simulink subsystem "out_of_wave"  (R2025b)
settings: Solver=VariableStepAuto  StartTime=0.0  StopTime=10.0  RelTol=1e-3
settings Model: Creator=sanborkl  LastModifiedBy=jdcjdb

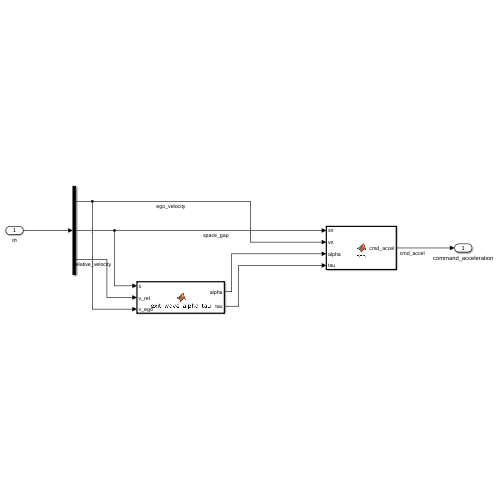
[thumbnail: Simulink's stored preview of the top-level diagram]
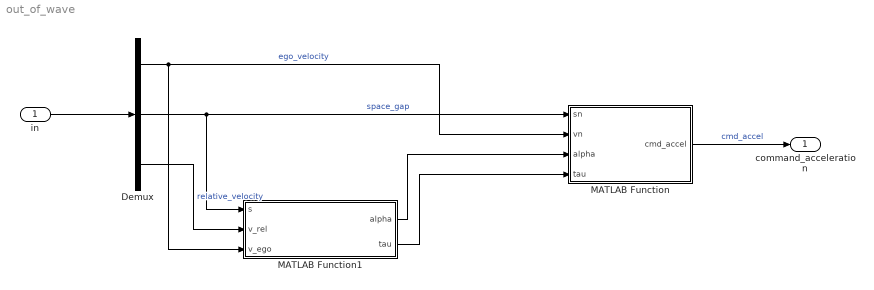
== system out_of_wave ==
  in : Inport
  Demux : Demux  Outputs=3
  MATLAB Function : MATLAB Function  TreatAsAtomicUnit=on
  MATLAB Function1 : MATLAB Function  TreatAsAtomicUnit=on
  command_acceleration : Outport
  wires:
  MATLAB Function1/1(alpha) -> MATLAB Function/3(alpha)
  MATLAB Function1/2(tau) -> MATLAB Function/4(tau)
  in/1 -> Demux/1
  Demux/1 -> MATLAB Function1/3(v_ego), MATLAB Function/2(vn)  "ego_velocity"
  Demux/2 -> MATLAB Function1/1(s), MATLAB Function/1(sn)  "space_gap"
  MATLAB Function/1(cmd_accel) -> command_acceleration/1  "cmd_accel"
  Demux/3 -> MATLAB Function1/2(v_rel)  "relative_velocity"

== matlab function out_of_wave/MATLAB Function1 ==
  data: s input; alpha output; v_rel input; v_ego input; tau output
function [alpha, tau] = exit_wave_alpha_tau(s, v_rel, v_ego)
%#codegen
% EXIT-WAVE: Decrease tau and increase alpha when the lead pulls away or gap is long.
% Inputs/Outputs same as Enter function.

% ===== Tunables =====
s0         = 2.0;    % [m]
tau_base   = 1.3;    % [s] base headway in Exit
tau_min    = 0.8;    % [s]
tau_max    = 2.0;    % [s]

alpha_base = 0.70;   % [-]
alpha_min  = 0.35;   % [-]
alpha_max  = 0.98;   % [-]

% Reactivity (pull-away / long-gap emphasis):
k_tau_relp = 0.06;   % [s^2/m]  tau -= k * (v_rel)+
k_tau_gapp = 0.03;   % [s/m]    tau -= k * (s - s_des0)+
k_a_relp   = 0.12;   % [-/(m/s)] alpha += k * (v_rel)+
k_a_gapp   = 0.03;   % [-/m]     alpha += k * (s - s_des0)+

% Smoothing
Ts         = 0.01;   % [s]
T_alpha    = 0.25;   % [s]
T_tau      = 0.25;   % [s]
% =====================

s_des0  = s0 + tau_base * v_ego;
pull    = max( v_rel, 0.0 );        % m/s (only when lead faster)
longgap = max( s - s_des0, 0.0 );   % m   (only when too far)

tau_tgt   = clamp(tau_base - k_tau_relp*pull - k_tau_gapp*longgap, tau_min,  tau_max);
alpha_tgt = clamp(alpha_base + k_a_relp*pull + k_a_gapp*longgap,   alpha_min, alpha_max);

persistent alpha_prev tau_prev
if isempty(alpha_prev); alpha_prev = alpha_tgt; end
if isempty(tau_prev);   tau_prev   = tau_tgt;   end

b_a = (T_alpha > 1e-6) * (Ts/(T_alpha+Ts)) + (T_alpha <= 1e-6) * 1.0;
b_t = (T_tau   > 1e-6) * (Ts/(T_tau  +Ts)) + (T_tau   <= 1e-6) * 1.0;

alpha = alpha_prev + b_a * (alpha_tgt - alpha_prev);
tau   = tau_prev   + b_t * (tau_tgt   - tau_prev);

alpha_prev = alpha;
tau_prev   = tau;

function y = clamp(x, lo, hi)
%#codegen
y = min(max(x, lo), hi);
end
end

== matlab function out_of_wave/MATLAB Function ==
  data: sn input; cmd_accel output; vn input; alpha input; tau input
function cmd_accel = fcn(sn, vn, alpha, tau)

cmd_accel = alpha * (sn - tau * vn);
